simulink model "differential_flatness_sim"  (R2017a)
settings: Solver=ode15s  StartTime=0.0  StopTime=10000  RelTol=1e-3  EnableMultiTasking=on
InitFcn:
  | param_quadrotor
undefined symbols (not defined in the file or in its folder): differential_flatness, drawDrone, Drone_Autopilot, forces_moments, P, plotstatevariables, true_states
libraries: simulink x3
settings Model: Creator=beard  LastModifiedBy=jacob
settings DataIOCC: LimitDataPoints=on  SaveFormat=Array  SignalLoggingSaveFormat=ModelDataLogs
settings OptimizationCC: ExpressionDepthLimit=2147483647  InitFltsAndDblsToZero=on  LifeSpan=inf
settings DebuggingCC: UnderspecifiedInitializationDetection=Classic  MergeDetectMultiDrivingBlocksExec=none  SolverPrmCheckMsg=warning  FcnCallInpInsideContextMsg=warning  StateNameClashWarn=warning  SFUnexpectedBacktrackingDiag=warning  SFNoUnconditionalDefaultTransitionDiag=warning  SFExecutionAtInitializationDiag=none
settings HardwareCC: ProdBitPerPointer=32  ProdBitPerSizeT=32  ProdBitPerPtrDiffT=32  ProdLargestAtomicFloat=None  ProdIntDivRoundTo=Undefined  ProdEndianess=Unspecified  ProdWordSize=32  ProdHWDeviceType=32-bit Generic
settings ModelReferenceCC: PropagateSignalLabelsOutOfModel=off
settings GRTTargetCC: TargetLangStandard=C89/C90 (ANSI)  GeneratePreprocessorConditionals=Disable all  CombineOutputUpdateFcns=off  GRTInterface=on
settings ConfigComp: CovMetricSettings=dw  CovHtmlReporting=on  CovSaveCumulativeToWorkspaceVar=on  CovSaveSingleToWorkspaceVar=on  CovExternalEMLEnable=off  CovSFcnEnable=off

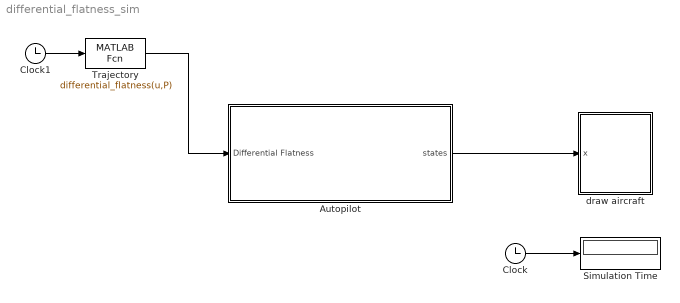
== system differential_flatness_sim ==
  Autopilot : Subsystem
  Clock : Clock
  Clock1 : Clock
  Simulation Time : Display
  Trajectory : MATLABFcn  MATLABFcn=differential_flatness(u,P)  OutputDimensions=11
  draw aircraft : Subsystem
  wires:
  Clock/1 -> Simulation Time/1
  Autopilot/1(states) -> draw aircraft/1(x)
  Clock1/1 -> Trajectory/1
  Trajectory/1 -> Autopilot/1(Differential Flatness)

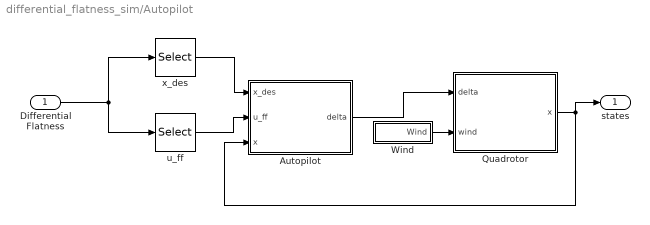
== system differential_flatness_sim/Autopilot ==
  Differential Flatness : Inport
  Autopilot : Subsystem
  Quadrotor : Subsystem
  Wind : Subsystem
  u_ff : Selector  InputPortWidth=11  IndexOptions=Index vector (dialog)  Indices=[8 9 10 11]  OutputSizes=1
  x_des : Selector  InputPortWidth=11  IndexOptions=Index vector (dialog)  Indices=[1 2 3 4 5 6 7]  OutputSizes=1
  states : Outport
  wires:
  Wind/1(Wind) -> Quadrotor/2(wind)
  Quadrotor/1(x) -> Autopilot/3(x), states/1
  Autopilot/1(delta) -> Quadrotor/1(delta)
  Differential Flatness/1 -> u_ff/1, x_des/1
  x_des/1 -> Autopilot/1(x_des)
  u_ff/1 -> Autopilot/2("u_ff ")

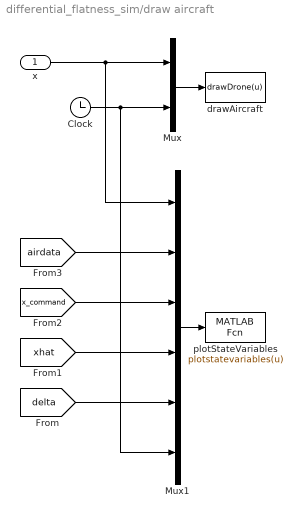
== system differential_flatness_sim/draw aircraft ==
  x : Inport
  Clock : Clock
  Mux : Mux  Inputs=2
  Mux1 : Mux  Inputs=6
  drawAircraft : MATLABFcn  MATLABFcn=drawDrone(u)  OutputDimensions=0  SampleTime=0.1
  plotStateVariables : MATLABFcn  MATLABFcn=plotstatevariables(u)  OutputDimensions=0  SampleTime=0.1
  wires:
  Mux/1 -> drawAircraft/1
  x/1 -> Mux/1, Mux1/1
  Clock/1 -> Mux/2, Mux1/6
  Mux1/1 -> plotStateVariables/1
  [xhat] -> Mux1/4
  [x_command] -> Mux1/3
  [delta] -> Mux1/5
  [airdata] -> Mux1/2

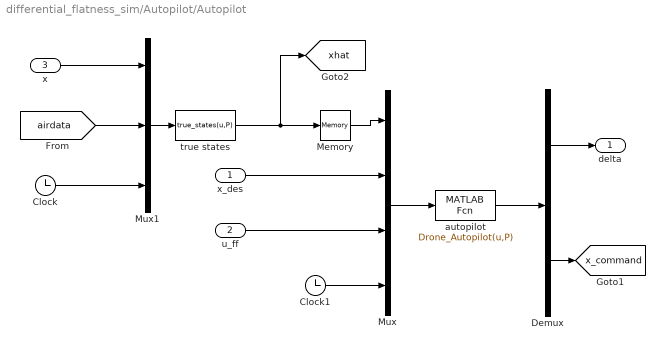
== system differential_flatness_sim/Autopilot/Autopilot ==
  x_des : Inport
  "u_ff " : Inport  Port=2
  x : Inport  Port=3
  Clock : Clock
  Clock1 : Clock
  Demux : Demux  Outputs=[4;12]
  Memory : Memory
  Mux : Mux
  Mux1 : Mux  Inputs=3
  autopilot : MATLABFcn  MATLABFcn=Drone_Autopilot(u,P)  OutputDimensions=4+12  SampleTime=P.Ts
  true states : MATLABFcn  MATLABFcn=true_states(u,P)  OutputDimensions=17  SampleTime=P.Ts
  delta : Outport
  tag scope: x_command=global, xhat=global
  wires:
  Mux/1 -> autopilot/1
  Clock/1 -> Mux1/3
  autopilot/1 -> Demux/1
  Demux/1 -> delta/1
  Demux/2 -> [x_command]
  x_des/1 -> Mux/2
  Mux1/1 -> true states/1
  x/1 -> Mux1/1
  true states/1 -> [xhat], Memory/1
  [airdata] -> Mux1/2
  Memory/1 -> Mux/1
  Clock1/1 -> Mux/4
  "u_ff "/1 -> Mux/3

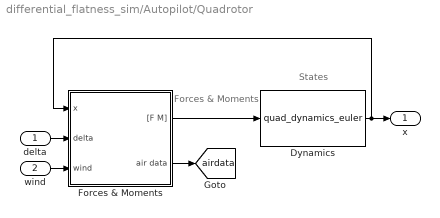
== system differential_flatness_sim/Autopilot/Quadrotor ==
  note: Forces & Moments
  note: States
  delta : Inport
  wind : Inport  Port=2
  Dynamics : S-Function  FunctionName=quad_dynamics_euler  Parameters=P  SFunctionDeploymentMode=off  EnableBusSupport=off
  Forces & Moments : Subsystem
  x : Outport
  tag scope: airdata=global
  wires:
  Dynamics/1 -> x/1, Forces & Moments/1(x)
  Forces & Moments/1("[F M]") -> Dynamics/1
  Forces & Moments/2(air data) -> [airdata]
  delta/1 -> Forces & Moments/2(delta)
  wind/1 -> Forces & Moments/3(wind)

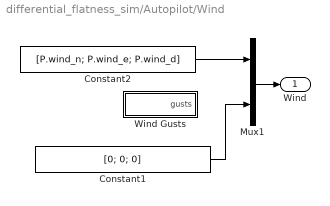
== system differential_flatness_sim/Autopilot/Wind ==
  Constant1 : Constant  Value=[0; 0; 0]
  Constant2 : Constant  Value=[P.wind_n; P.wind_e; P.wind_d]
  Mux1 : Mux  Inputs=2
  Wind Gusts : Subsystem
  Wind : Outport
  wires:
  Constant2/1 -> Mux1/1
  Mux1/1 -> Wind/1
  Constant1/1 -> Mux1/2

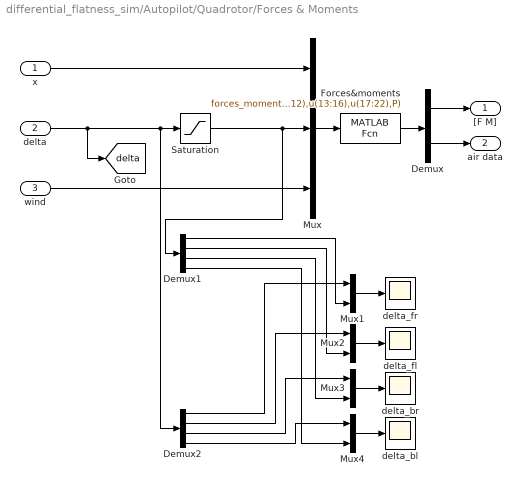
== system differential_flatness_sim/Autopilot/Quadrotor/Forces & Moments ==
  x : Inport
  delta : Inport  Port=2
  wind : Inport  Port=3
  Demux : Demux  Outputs=[6;6]
  Demux1 : Demux
  Demux2 : Demux
  Forces&moments : MATLABFcn  MATLABFcn=forces_moments(u(1:12),u(13:16),u(17:22),P)  OutputDimensions=12
  Mux : Mux  Inputs=3
  Mux{1..4} (4 alike) : Mux  Inputs=2
  Saturation : Saturate  UpperLimit=1  LowerLimit=0
  delta_bl : Scope
  delta_br : Scope
  delta_fl : Scope
  delta_fr : Scope
  "[F M]" : Outport
  air data : Outport  Port=2
  tag scope: delta=global
  wires:
  Demux/2 -> air data/1
  Mux/1 -> Forces&moments/1
  Demux/1 -> "[F M]"/1
  Forces&moments/1 -> Demux/1
  wind/1 -> Mux/3
  delta/1 -> Demux2/1, Saturation/1, [delta]
  x/1 -> Mux/1
  Saturation/1 -> Demux1/1, Mux/2
  Mux1/1 -> delta_fr/1
  Demux1/1 -> Mux1/2
  Demux2/1 -> Mux1/1
  Mux2/1 -> delta_fl/1
  Mux3/1 -> delta_br/1
  Mux4/1 -> delta_bl/1
  Demux1/4 -> Mux4/2
  Demux1/2 -> Mux2/2
  Demux1/3 -> Mux3/2
  Demux2/2 -> Mux2/1
  Demux2/3 -> Mux3/1
  Demux2/4 -> Mux4/1

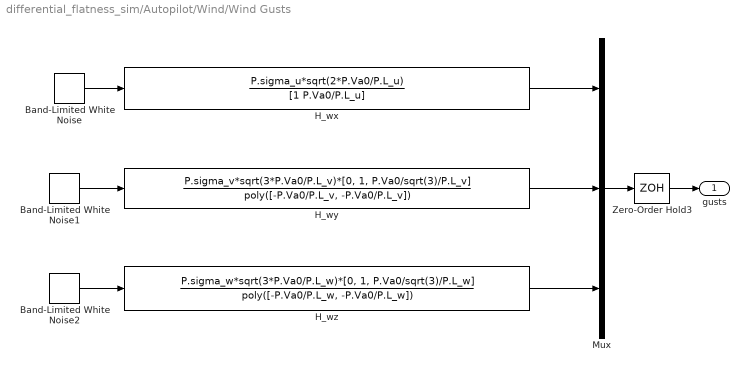
== system differential_flatness_sim/Autopilot/Wind/Wind Gusts ==
  Band-Limited White Noise : simulink/Sources/Band-Limited White Noise  Cov=[1]  Ts=P.Ts  seed=[23341]
  Band-Limited White Noise1 : simulink/Sources/Band-Limited White Noise  Cov=[1]  Ts=P.Ts  seed=[23341]
  Band-Limited White Noise2 : simulink/Sources/Band-Limited White Noise  Cov=[1]  Ts=P.Ts  seed=[23341]
  H_wx : TransferFcn  Numerator=P.sigma_u*sqrt(2*P.Va0/P.L_u)  Denominator=[1 P.Va0/P.L_u]
  H_wy : TransferFcn  Numerator=P.sigma_v*sqrt(3*P.Va0/P.L_v)*[0, 1, P.Va0/sqrt(3)/P.L_v]  Denominator=poly([-P.Va0/P.L_v, -P.Va0/P.L_v])
  H_wz : TransferFcn  Numerator=P.sigma_w*sqrt(3*P.Va0/P.L_w)*[0, 1, P.Va0/sqrt(3)/P.L_w]  Denominator=poly([-P.Va0/P.L_w, -P.Va0/P.L_w])
  Mux : Mux  Inputs=3
  Zero-Order Hold3 : ZeroOrderHold  SampleTime=P.Ts
  gusts : Outport
  wires:
  H_wx/1 -> Mux/1
  Band-Limited White Noise/1 -> H_wx/1
  H_wy/1 -> Mux/2
  Band-Limited White Noise1/1 -> H_wy/1
  H_wz/1 -> Mux/3
  Band-Limited White Noise2/1 -> H_wz/1
  Mux/1 -> Zero-Order Hold3/1
  Zero-Order Hold3/1 -> gusts/1
